simulink model "ControlSystem_Simlulation"  (R2021a)
settings: Solver=VariableStepAuto  StartTime=0.0  StopTime=20  FixedStep=0.05  RelTol=1e-3
undefined symbols (not defined in the file or in its folder): DiscIntNeverNeededParam
libraries: simulink x2, simulink_extras x2, shared6dof x1, aerolibanimutils x1
settings Model: SimulationMode=external  SILPILModeSetting=veronly  ExtModeTrigDuration=2  Creator=Samsung  LastModifiedBy=Samsung
settings SolverCC: AutoInsertRateTranBlk=on
settings OptimizationCC: DefaultParameterBehavior=Inlined  EnhancedBackFolding=on  PassReuseOutputArgsThreshold=0  MaxStackSize=64  OptimizeBlockOrder=speed  DifferentSizesBufferReuse=on  OptimizationCustomize=off
settings DebuggingCC: ParameterTunabilityLossMsg=error
settings HardwareCC: ProdHWDeviceType=AMD->x86-64 (Windows64)  TargetBitPerPointer=64  TargetBitPerSizeT=64  TargetBitPerPtrDiffT=64  TargetLongLongMode=on  TargetIntDivRoundTo=Zero  TargetEndianess=LittleEndian  TargetWordSize=64  TargetHWDeviceType=MATLAB Host  ProdEqTarget=off
settings SFSimCC: MATLABDynamicMemAlloc=off
settings RTWCC: Description=Rapid Simulation Target  SystemTargetFile=rsim.tlc  TemplateMakefile=rsim_default_tmf  Toolchain=Arduino ARM MBED  BuildConfiguration=Faster Runs
settings CodeAppCC: ForceParamTrailComments=on  OperatorAnnotations=on

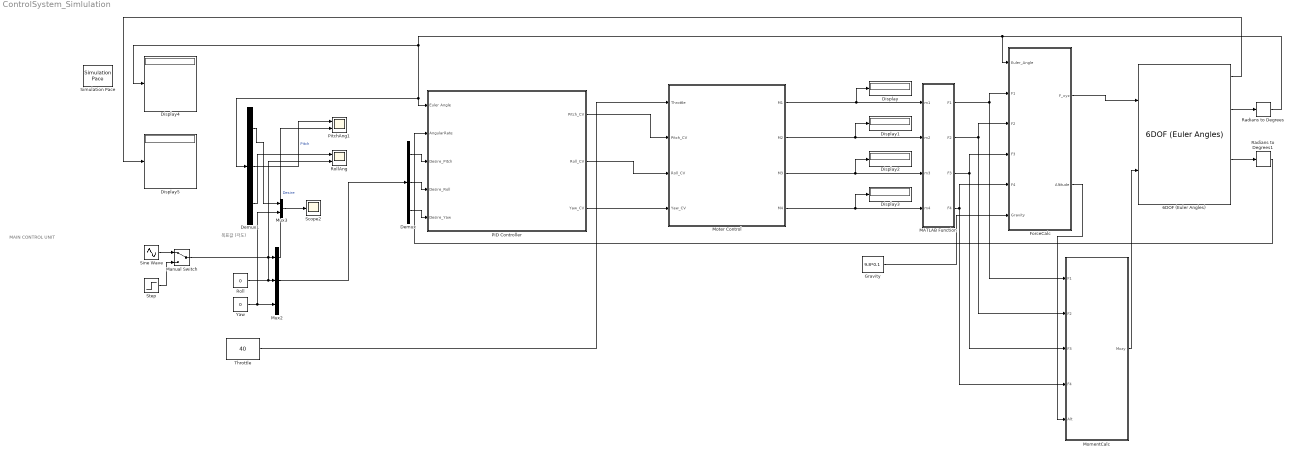
== system ControlSystem_Simlulation ==
  note: MAIN CONTROL UNIT
  note: 목표값 (각도)
  6DOF (Euler Angles) : shared6dof/6DOF (Euler Angles)  units=Metric (MKS)  mtype=Fixed  rep=Euler Angles  xme_0=[0 0 0]  Vm_0=[0 0 0]  eul_0=[0 0 0]  pm_0=[0 0 0]  mass_0=1  mass_e=0.5  mass_f=2.0  inertia=[0.1 0 0; 0 0.1 0; 0 0 0.2;]  inertia_e=eye(3)  inertia_f=2*eye(3)  k_quat=1.0  vre_flag=on  abi_flag=off  aMode=0  xme_statename=''  Vm_statename=''  eul_statename=''  quat_statename=''  pm_statename=''  mass_statename=''
      settings: SourceProductBaseCode=AE,PW,DR,MT,UV,VE
  Demux : Demux  Outputs=3
  Demux1 : Demux  Outputs=3
  Display{,1..5} (6 alike) : Display
  ForceCalc : Subsystem
  Gravity : Constant  Value=9.8*0.1
  MATLAB Function : MATLAB Function  TreatAsAtomicUnit=on
  Manual Switch : ManualSwitch
  MomentCalc : Subsystem
  Moter Control : Subsystem
  Mux2 : Mux  Inputs=3
  Mux3 : Mux  Inputs=2
  PID Controller : Subsystem
  PitchAng1 : Scope  NumInputPorts=2
  Radians to Degrees : simulink_extras/Transformations/Radians to Degrees
  Radians to Degrees1 : simulink_extras/Transformations/Radians to Degrees
  Roll : Constant  Value=0
  RollAng : Scope  NumInputPorts=2
  Scope2 : Scope
  Simulation Pace : aerolibanimutils/Simulation Pace  SimulationPace=2  SleepMode=Auto  OutputPaceError=off  SampleTime=1/30
  Sine Wave : Sin  Amplitude=10  Bias=10  SampleTime=0
  Step : Step  After=10  SampleTime=0
  Throttle : Constant  Value=40
  Yaw : Constant  Value=0
  wires:
  PID Controller/1(Pitch_CV) -> Moter Control/2(Pitch_CV)
  PID Controller/2(Roll_CV) -> Moter Control/3(Roll_CV)
  PID Controller/3(Yaw_CV) -> Moter Control/4(Yaw_CV)
  Roll/1 -> RollAng/2, Mux2/2
  Yaw/1 -> Mux3/2, Mux2/3
  Demux/2 -> PID Controller/4(Desire_Roll)
  Demux/1 -> PID Controller/3(Desire_Pitch)
  Demux/3 -> PID Controller/5(Desire_Yaw)
  Mux2/1 -> Demux/1
  Throttle/1 -> Moter Control/1(Throttle)
  Moter Control/4(M4) -> Display3/1, MATLAB Function/4(m4)
  Moter Control/3(M3) -> Display2/1, MATLAB Function/3(m3)
  Moter Control/2(M2) -> Display1/1, MATLAB Function/2(m2)
  Moter Control/1(M1) -> Display/1, MATLAB Function/1(m1)
  MATLAB Function/1(F1) -> ForceCalc/2(F1), MomentCalc/1(F1)
  MATLAB Function/2(F2) -> ForceCalc/3(F2), MomentCalc/2(F2)
  MATLAB Function/3(F3) -> ForceCalc/4(F3), MomentCalc/3(F3)
  MATLAB Function/4(F4) -> ForceCalc/5(F4), MomentCalc/4(F4)
  ForceCalc/1(F_xyz) -> 6DOF (Euler Angles)/1
  MomentCalc/1(Mxzy) -> 6DOF (Euler Angles)/2
  Mux3/1 -> Scope2/1
  6DOF (Euler Angles)/3 -> Radians to Degrees/1
  6DOF (Euler Angles)/6 -> Radians to Degrees1/1
  Radians to Degrees/1 -> ForceCalc/1(Euler_Angle), Demux1/1, PID Controller/1(Euler Angle), Display4/1
  Radians to Degrees1/1 -> PID Controller/2(AngularRate)
  Demux1/2 -> PitchAng1/1  "Pitch"
  Demux1/3 -> RollAng/1
  Demux1/1 -> Mux3/1
  6DOF (Euler Angles)/1 -> Display5/1
  Manual Switch/1 -> PitchAng1/2, Mux2/1  "Desire"
  Sine Wave/1 -> Manual Switch/1
  Step/1 -> Manual Switch/2
  Gravity/1 -> ForceCalc/6(Gravity)
  ForceCalc/2(Altitude) -> MomentCalc/5(Alt)

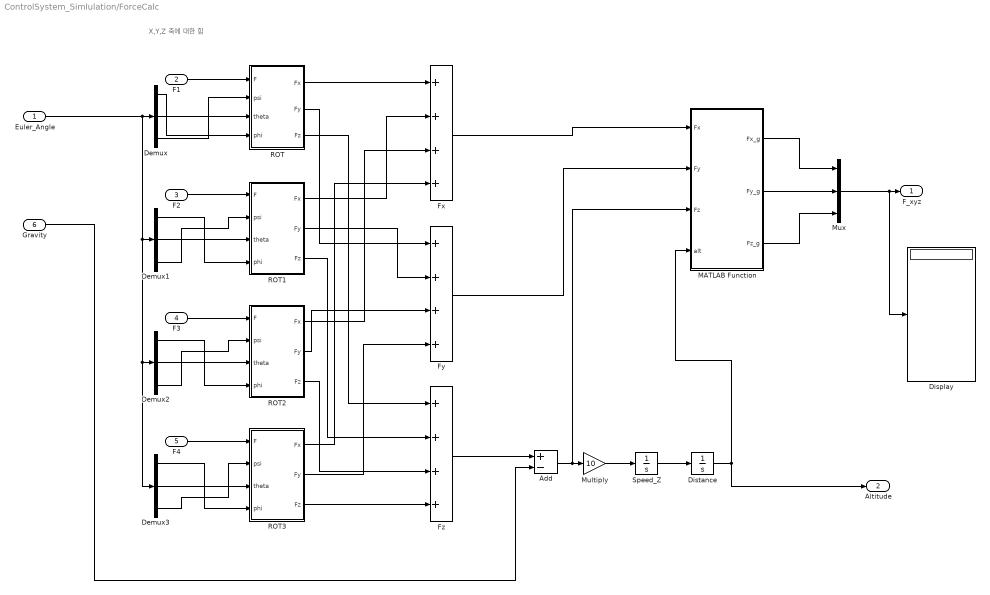
== system ControlSystem_Simlulation/ForceCalc ==
  note: X,Y,Z 축에 대한 힘
  Euler_Angle : Inport
  F1 : Inport  Port=2
  F2 : Inport  Port=3
  F3 : Inport  Port=4
  F4 : Inport  Port=5
  Gravity : Inport  Port=6
  Add : Sum  Inputs=+-
  Demux{,1..3} (4 alike) : Demux  Outputs=3
  Display : Display
  Distance : Integrator
  Fx : Sum  Inputs=++++
  Fy : Sum  Inputs=++++
  Fz : Sum  Inputs=++++
  MATLAB Function : MATLAB Function  TreatAsAtomicUnit=on
  Multiply : Gain  Gain=10
  Mux : Mux  Inputs=3
  ROT : MATLAB Function  TreatAsAtomicUnit=on
  ROT1 : MATLAB Function  TreatAsAtomicUnit=on
  ROT2 : MATLAB Function  TreatAsAtomicUnit=on
  ROT3 : MATLAB Function  TreatAsAtomicUnit=on
  Speed_Z : Integrator
  F_xyz : Outport
  Altitude : Outport  Port=2
  wires:
  Euler_Angle/1 -> Demux/1, Demux3/1, Demux2/1, Demux1/1
  Demux/2 -> ROT/3(theta)
  F1/1 -> ROT/1(F)
  F2/1 -> ROT1/1(F)
  Demux1/2 -> ROT1/3(theta)
  Demux2/2 -> ROT2/3(theta)
  F3/1 -> ROT2/1(F)
  Demux3/2 -> ROT3/3(theta)
  F4/1 -> ROT3/1(F)
  ROT/1(Fx) -> Fx/1
  ROT1/1(Fx) -> Fx/2
  ROT2/1(Fx) -> Fx/3
  ROT3/1(Fx) -> Fx/4
  ROT/2(Fy) -> Fy/1
  ROT1/2(Fy) -> Fy/2
  ROT2/2(Fy) -> Fy/3
  ROT3/2(Fy) -> Fy/4
  ROT/3(Fz) -> Fz/1
  ROT1/3(Fz) -> Fz/2
  ROT2/3(Fz) -> Fz/3
  ROT3/3(Fz) -> Fz/4
  Mux/1 -> Display/1, F_xyz/1
  Demux/1 -> ROT/4(phi)
  Demux/3 -> ROT/2(psi)
  Demux1/1 -> ROT1/4(phi)
  Demux1/3 -> ROT1/2(psi)
  Demux2/1 -> ROT2/4(phi)
  Demux2/3 -> ROT2/2(psi)
  Demux3/1 -> ROT3/4(phi)
  Demux3/3 -> ROT3/2(psi)
  Fz/1 -> Add/1
  Gravity/1 -> Add/2
  Add/1 -> MATLAB Function/3(Fz), Multiply/1
  Multiply/1 -> Speed_Z/1
  Speed_Z/1 -> Distance/1
  MATLAB Function/2(Fy_g) -> Mux/2
  MATLAB Function/1(Fx_g) -> Mux/1
  MATLAB Function/3(Fz_g) -> Mux/3
  Distance/1 -> Altitude/1, MATLAB Function/4(alt)
  Fy/1 -> MATLAB Function/2(Fy)
  Fx/1 -> MATLAB Function/1(Fx)

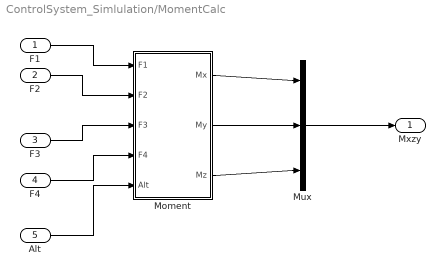
== system ControlSystem_Simlulation/MomentCalc ==
  F1 : Inport
  F2 : Inport  Port=2
  F3 : Inport  Port=3
  F4 : Inport  Port=4
  Alt : Inport  Port=5
  Moment : MATLAB Function  TreatAsAtomicUnit=on
  Mux : Mux  Inputs=3
  Mxzy : Outport
  wires:
  F1/1 -> Moment/1(F1)
  F2/1 -> Moment/2(F2)
  F3/1 -> Moment/3(F3)
  F4/1 -> Moment/4(F4)
  Moment/1(Mx) -> Mux/1
  Moment/2(My) -> Mux/2
  Moment/3(Mz) -> Mux/3
  Mux/1 -> Mxzy/1
  Alt/1 -> Moment/5(Alt)

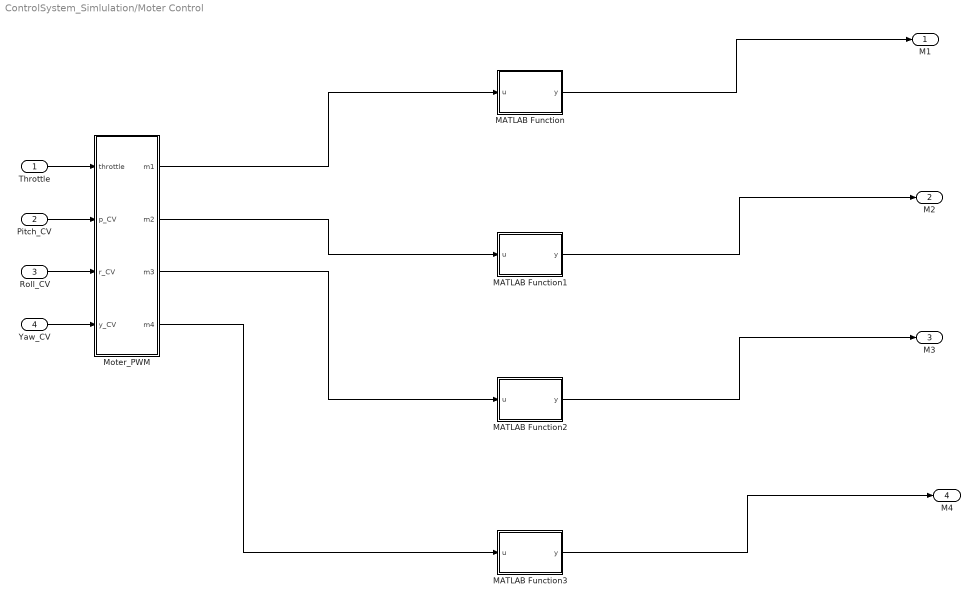
== system ControlSystem_Simlulation/Moter Control ==
  Throttle : Inport
  Pitch_CV : Inport  Port=2
  Roll_CV : Inport  Port=3
  Yaw_CV : Inport  Port=4
  MATLAB Function : MATLAB Function  TreatAsAtomicUnit=on
  MATLAB Function1 : MATLAB Function  TreatAsAtomicUnit=on
  MATLAB Function2 : MATLAB Function  TreatAsAtomicUnit=on
  MATLAB Function3 : MATLAB Function  TreatAsAtomicUnit=on
  Moter_PWM : MATLAB Function  TreatAsAtomicUnit=on
  M1 : Outport
  M2 : Outport  Port=2
  M3 : Outport  Port=3
  M4 : Outport  Port=4
  wires:
  Moter_PWM/1(m1) -> MATLAB Function/1(u)
  Moter_PWM/2(m2) -> MATLAB Function1/1(u)
  Moter_PWM/3(m3) -> MATLAB Function2/1(u)
  Moter_PWM/4(m4) -> MATLAB Function3/1(u)
  Throttle/1 -> Moter_PWM/1(throttle)
  Pitch_CV/1 -> Moter_PWM/2(p_CV)
  Roll_CV/1 -> Moter_PWM/3(r_CV)
  Yaw_CV/1 -> Moter_PWM/4(y_CV)
  MATLAB Function/1(y) -> M1/1
  MATLAB Function1/1(y) -> M2/1
  MATLAB Function2/1(y) -> M3/1
  MATLAB Function3/1(y) -> M4/1

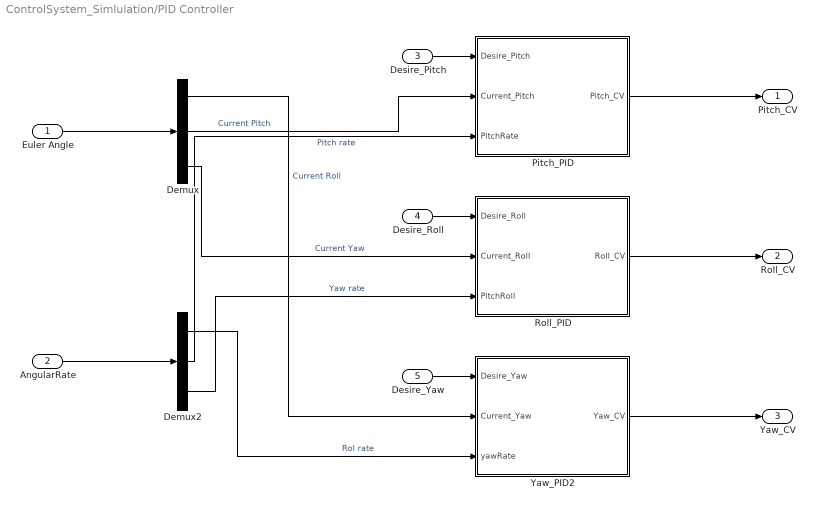
== system ControlSystem_Simlulation/PID Controller ==
  Euler Angle : Inport
  AngularRate : Inport  Port=2
  Desire_Pitch : Inport  Port=3
  Desire_Roll : Inport  Port=4
  Desire_Yaw : Inport  Port=5
  Demux : Demux  Outputs=3
  Demux2 : Demux  Outputs=3
  Pitch_PID : Subsystem
  Roll_PID : Subsystem
  Yaw_PID2 : Subsystem
  Pitch_CV : Outport
  Roll_CV : Outport  Port=2
  Yaw_CV : Outport  Port=3
  wires:
  Desire_Pitch/1 -> Pitch_PID/1(Desire_Pitch)
  Desire_Yaw/1 -> Yaw_PID2/1(Desire_Yaw)
  Pitch_PID/1(Pitch_CV) -> Pitch_CV/1
  Roll_PID/1(Roll_CV) -> Roll_CV/1
  Yaw_PID2/1(Yaw_CV) -> Yaw_CV/1
  Desire_Roll/1 -> Roll_PID/1(Desire_Roll)
  Demux/2 -> Pitch_PID/2(Current_Pitch)  "Current Pitch"
  Euler Angle/1 -> Demux/1
  AngularRate/1 -> Demux2/1
  Demux/1 -> Yaw_PID2/2(Current_Yaw)  "Current Roll"
  Demux/3 -> Roll_PID/2(Current_Roll)  "Current Yaw"
  Demux2/1 -> Yaw_PID2/3(yawRate)  "Rol rate"
  Demux2/2 -> Pitch_PID/3(PitchRate)  "Pitch rate"
  Demux2/3 -> Roll_PID/3(PitchRoll)  "Yaw rate"

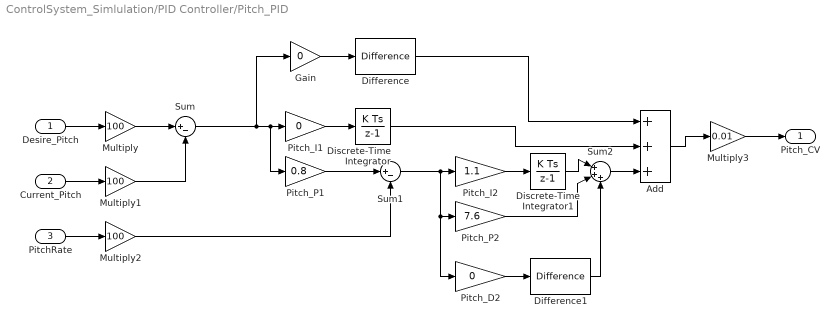
== system ControlSystem_Simlulation/PID Controller/Pitch_PID ==
  Desire_Pitch : Inport
  Current_Pitch : Inport  Port=2
  PitchRate : Inport  Port=3
  Add : Sum  Inputs=+++
  Difference : simulink/Discrete/Difference  ICPrevInput=0.0  OutMin=[]  OutMax=[]  OutDataType=fixdt(1, 16)  OutScaling=2^-10  DoSatur=off
  Difference1 : simulink/Discrete/Difference  ICPrevInput=0.0  OutMin=[]  OutMax=[]  OutDataType=fixdt(1, 16)  OutScaling=2^-10  DoSatur=off
  Discrete-Time Integrator : DiscreteIntegrator  SampleTime=-1  ICPrevOutput=DiscIntNeverNeededParam  ICPrevScaledInput=DiscIntNeverNeededParam
  Discrete-Time Integrator1 : DiscreteIntegrator  SampleTime=-1  ICPrevOutput=DiscIntNeverNeededParam  ICPrevScaledInput=DiscIntNeverNeededParam
  Gain : Gain  Gain=0
  Multiply : Gain  Gain=100
  Multiply1 : Gain  Gain=100
  Multiply2 : Gain  Gain=100
  Multiply3 : Gain  Gain=0.01
  Pitch_D2 : Gain  Gain=0
  Pitch_I1 : Gain  Gain=0
  Pitch_I2 : Gain  Gain=1.1
  Pitch_P1 : Gain  Gain=0.8
  Pitch_P2 : Gain  Gain=7.6
  Sum : Sum  Inputs=|+-
  Sum1 : Sum  Inputs=|+-
  Sum2 : Sum  Inputs=|+++
  Pitch_CV : Outport
  wires:
  Desire_Pitch/1 -> Multiply/1
  Current_Pitch/1 -> Multiply1/1
  Sum/1 -> Gain/1, Pitch_P1/1, Pitch_I1/1
  Pitch_I1/1 -> Discrete-Time Integrator/1
  Pitch_P1/1 -> Sum1/1
  PitchRate/1 -> Multiply2/1
  Sum1/1 -> Pitch_D2/1, Pitch_P2/1, Pitch_I2/1
  Pitch_I2/1 -> Discrete-Time Integrator1/1
  Pitch_P2/1 -> Sum2/2
  Discrete-Time Integrator1/1 -> Sum2/1
  Multiply/1 -> Sum/1
  Multiply1/1 -> Sum/2
  Multiply2/1 -> Sum1/2
  Add/1 -> Multiply3/1
  Multiply3/1 -> Pitch_CV/1
  Gain/1 -> Difference/1
  Sum2/1 -> Add/3
  Discrete-Time Integrator/1 -> Add/2
  Difference/1 -> Add/1
  Pitch_D2/1 -> Difference1/1
  Difference1/1 -> Sum2/3

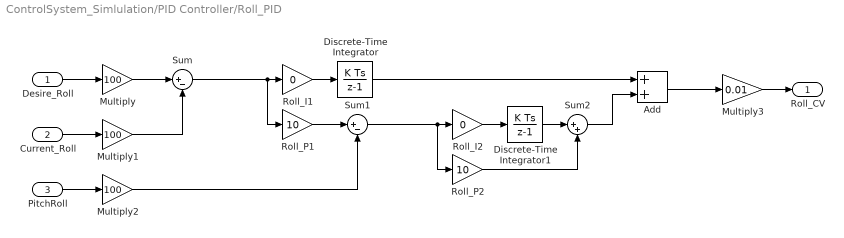
== system ControlSystem_Simlulation/PID Controller/Roll_PID ==
  Desire_Roll : Inport
  Current_Roll : Inport  Port=2
  PitchRoll : Inport  Port=3
  Add : Sum
  Discrete-Time Integrator : DiscreteIntegrator  SampleTime=-1  ICPrevOutput=DiscIntNeverNeededParam  ICPrevScaledInput=DiscIntNeverNeededParam
  Discrete-Time Integrator1 : DiscreteIntegrator  SampleTime=-1  ICPrevOutput=DiscIntNeverNeededParam  ICPrevScaledInput=DiscIntNeverNeededParam
  Multiply : Gain  Gain=100
  Multiply1 : Gain  Gain=100
  Multiply2 : Gain  Gain=100
  Multiply3 : Gain  Gain=0.01
  Roll_I1 : Gain  Gain=0
  Roll_I2 : Gain  Gain=0
  Roll_P1 : Gain  Gain=10
  Roll_P2 : Gain  Gain=10
  Sum : Sum  Inputs=|+-
  Sum1 : Sum  Inputs=|+-
  Sum2 : Sum  Inputs=|++
  Roll_CV : Outport
  wires:
  Roll_P2/1 -> Sum2/2
  Sum1/1 -> Roll_P2/1, Roll_I2/1
  Roll_I2/1 -> Discrete-Time Integrator1/1
  Discrete-Time Integrator1/1 -> Sum2/1
  Discrete-Time Integrator/1 -> Add/1
  Sum/1 -> Roll_P1/1, Roll_I1/1
  Sum2/1 -> Add/2
  Desire_Roll/1 -> Multiply/1
  PitchRoll/1 -> Multiply2/1
  Roll_P1/1 -> Sum1/1
  Current_Roll/1 -> Multiply1/1
  Roll_I1/1 -> Discrete-Time Integrator/1
  Add/1 -> Multiply3/1
  Multiply/1 -> Sum/1
  Multiply1/1 -> Sum/2
  Multiply2/1 -> Sum1/2
  Multiply3/1 -> Roll_CV/1

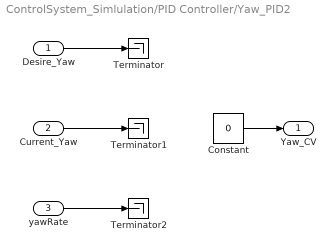
== system ControlSystem_Simlulation/PID Controller/Yaw_PID2 ==
  Desire_Yaw : Inport
  Current_Yaw : Inport  Port=2
  yawRate : Inport  Port=3
  Constant : Constant  Value=0
  Terminator : Terminator
  Terminator1 : Terminator
  Terminator2 : Terminator
  Yaw_CV : Outport
  wires:
  Desire_Yaw/1 -> Terminator/1
  Current_Yaw/1 -> Terminator1/1
  yawRate/1 -> Terminator2/1
  Constant/1 -> Yaw_CV/1

== matlab function ControlSystem_Simlulation/ForceCalc/ROT2 ==
  data: F input; psi input; theta input; Fx output; phi input; Fy output; Fz output
function [Fx, Fy, Fz] = ROT(F,psi,theta,phi)
% 회전행렬로 드론 추력을 좌표축에 대한 추력으로 변환
initThrust = [0; 0; F];

Z = [cosd(phi) -sind(phi) 0; sind(phi) cosd(phi) 0; 0 0 1] * initThrust;
Y = [cosd(theta) 0 -sind(theta); 0 1 0; sind(theta) 0 cosd(theta)] * initThrust;
X = [1 0 0; 0 cosd(psi) -sind(psi); 0 sind(psi) cosd(psi)] * initThrust;

result = X + Y + Z;
Fx = result(1);
Fy = result(2);
Fz = result(3);

== matlab function ControlSystem_Simlulation/ForceCalc/ROT3 ==
  data: F input; psi input; theta input; Fx output; phi input; Fy output; Fz output
function [Fx, Fy, Fz] = ROT(F,psi,theta,phi)
% 회전행렬로 드론 추력을 좌표축에 대한 추력으로 변환
initThrust = [0; 0; F];

Z = [cosd(phi) -sind(phi) 0; sind(phi) cosd(phi) 0; 0 0 1] * initThrust;
Y = [cosd(theta) 0 -sind(theta); 0 1 0; sind(theta) 0 cosd(theta)] * initThrust;
X = [1 0 0; 0 cosd(psi) -sind(psi); 0 sind(psi) cosd(psi)] * initThrust;


result = X + Y + Z;
Fx = result(1);
Fy = result(2);
Fz = result(3);

== matlab function ControlSystem_Simlulation/MomentCalc/Moment ==
  data: F1 input; Mx output; F2 input; F3 input; F4 input; My output; Mz output; Alt input
function [Mx,My,Mz] = Moments(F1,F2,F3,F4, Alt)
% 드론의 모멘트 계산
if Alt <= 0.3
    Mx = 0;
    My = 0;
    Mz = 0;
    
else
Mx = ((F1+F3)-(F2+F4))*0.08;
My = ((F2+F1)-(F4+F3))*0.08;
Mz = 0;
end

== matlab function ControlSystem_Simlulation/ForceCalc/MATLAB Function ==
  data: Fx input; Fx_g output; Fy input; Fz input; alt input; Fy_g output; Fz_g output
function [Fx_g,Fy_g,Fz_g] = fcn(Fx, Fy, Fz, alt)

% 지면 효과

if alt <= 0.3
    Fx_g = 0;
    Fy_g = 0;
    Fz_g = 0;

else

Fx_g = Fx;
Fy_g = Fy;
Fz_g = Fz;
end

== matlab function ControlSystem_Simlulation/Moter Control/MATLAB Function ==
  data: u input; y output
function y = IsUnderZero(u)
if u < 0
    u = 0;
end

y = u;

== matlab function ControlSystem_Simlulation/Moter Control/MATLAB Function1 ==
  data: u input; y output
function y = IsUnderZero(u)
if u < 0
    u = 0;
end

    y = u;

== matlab function ControlSystem_Simlulation/Moter Control/MATLAB Function2 ==
  data: u input; y output
function y = IsUnderZero(u)
if u < 0
    u = 0;
end

    y = u;

== matlab function ControlSystem_Simlulation/Moter Control/MATLAB Function3 ==
  data: u input; y output
function y = IsUnderZero(u)
if u < 0
    u = 0;
end

    y = u;

== matlab function ControlSystem_Simlulation/Moter Control/Moter_PWM ==
  data: throttle input; m1 output; p_CV input; r_CV input; y_CV input; m2 output; m3 output; m4 output
function [m1, m2, m3, m4] = MoterPWM(throttle, p_CV, r_CV, y_CV)

if throttle == 0
    m1 = 0;
    m2 = 0;
    m3 = 0;
    m4 = 0;

else
    m2 = throttle + p_CV + r_CV + y_CV;
    m4 = throttle - p_CV + r_CV - y_CV;
    m1 = throttle + p_CV - r_CV - y_CV;
    m3 = throttle - p_CV - r_CV + y_CV;
end

== matlab function ControlSystem_Simlulation/MATLAB Function ==
  data: m1 input; F1 output; m2 input; m3 input; m4 input; F2 output; F3 output; F4 output
function [F1,F2,F3,F4] = pwm2force(m1,m2,m3,m4)
% PWM 에 따른 모터 힘
% 실험을 통해 측정

% 255 -> 30g 추력 으로 가정, 0 ~ 255 는 선형
% 3.7v 일때 기준
% 출력단위는 N
% 따라서 255 일때 0.294N
MAX_THRUST = 0.294;

F1 = MAX_THRUST * (m1/255);
F2 = MAX_THRUST * (m2/255);
F3 = MAX_THRUST * (m3/255);
F4 = MAX_THRUST * (m4/255);

== matlab function ControlSystem_Simlulation/ForceCalc/ROT ==
  data: F input; psi input; theta input; Fx output; phi input; Fy output; Fz output
function [Fx, Fy, Fz] = ROT(F,psi,theta,phi)
% 회전행렬로 드론 추력을 좌표축에 대한 추력으로 변환
initThrust = [0; 0; F];

Z = [cosd(phi) -sind(phi) 0; sind(phi) cosd(phi) 0; 0 0 1] * initThrust;
Y = [cosd(theta) 0 -sind(theta); 0 1 0; sind(theta) 0 cosd(theta)] * initThrust;
X = [1 0 0; 0 cosd(psi) -sind(psi); 0 sind(psi) cosd(psi)] * initThrust;

result = X + Y + Z;
Fx = result(1);
Fy = result(2);
Fz = result(3);

== matlab function ControlSystem_Simlulation/ForceCalc/ROT1 ==
  data: F input; psi input; theta input; Fx output; phi input; Fy output; Fz output
function [Fx, Fy, Fz] = ROT(F,psi,theta,phi)
% 회전행렬로 드론 추력을 좌표축에 대한 추력으로 변환
initThrust = [0; 0; F];

Z = [cosd(phi) -sind(phi) 0; sind(phi) cosd(phi) 0; 0 0 1] * initThrust;
Y = [cosd(theta) 0 -sind(theta); 0 1 0; sind(theta) 0 cosd(theta)] * initThrust;
X = [1 0 0; 0 cosd(psi) -sind(psi); 0 sind(psi) cosd(psi)] * initThrust;

result = X + Y + Z;
Fx = result(1);
Fy = result(2);
Fz = result(3);
